simulink model ""  (R2025b)
settings: Solver=FixedStepAuto  StartTime=0.0  StopTime=inf  FixedStep=.02  RelTol=1e-3
libraries: simulink x3
settings Model: Creator=ajax  LastModifiedBy=ajax

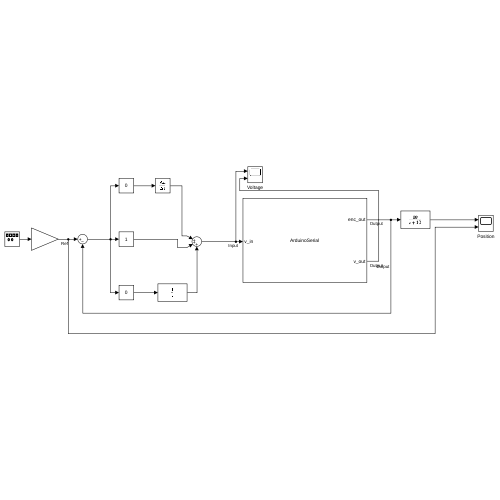
[thumbnail: Simulink's stored preview of the top-level diagram]
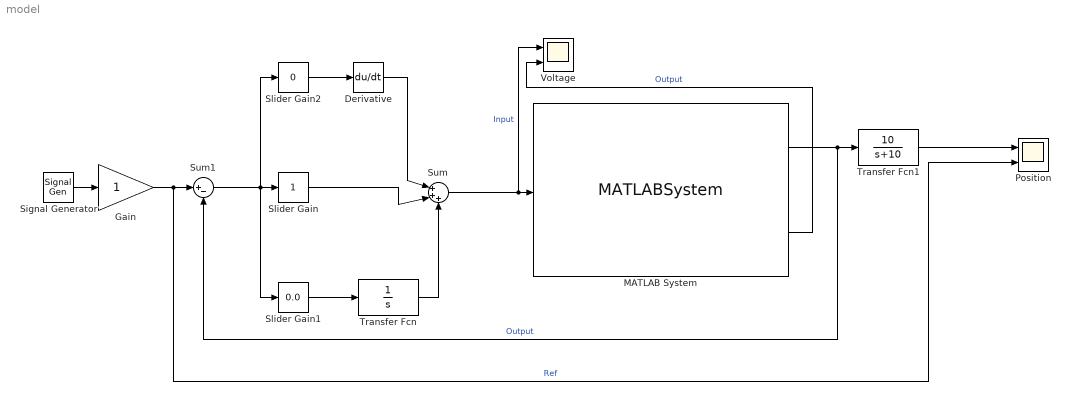
== system model ==
  Derivative : Derivative
  Gain : Gain
  MATLAB System : MATLABSystem  System=ArduinoSerial  COMPort=/dev/ttyACM0  BaudRate=115200  SimulateUsing=Interpreted execution
      mask Type: ArduinoSerial
  Position : Scope  NumInputPorts=2
      settings: ActiveDisplayYMinimum=-12131.749999999998  ActiveDisplayYMaximum=109165.75
  Signal Generator : SignalGenerator  WaveForm=square  Frequency=.5
  Slider Gain : simulink/Math Operations/Slider Gain  gain=1  low=0  high=2
  Slider Gain1 : simulink/Math Operations/Slider Gain  gain=0.0  low=0  high=2
  Slider Gain2 : simulink/Math Operations/Slider Gain  gain=0  low=0  high=2
  Sum : Sum  Inputs=|+++
  Sum1 : Sum  Inputs=|+-
  Transfer Fcn : TransferFcn  Denominator=[1 0]
  Transfer Fcn1 : TransferFcn  Numerator=[10]  Denominator=[1 10]
  Voltage : Scope  NumInputPorts=2
      settings: ActiveDisplayYMinimum=-108237.6717  ActiveDisplayYMaximum=3759.045299999998
  wires:
  Slider Gain2/1 -> Derivative/1
  Derivative/1 -> Sum/1
  Slider Gain/1 -> Sum/2
  Slider Gain1/1 -> Transfer Fcn/1
  Transfer Fcn/1 -> Sum/3
  MATLAB System/1 -> Transfer Fcn1/1, Sum1/2  "Output"
  Signal Generator/1 -> Gain/1
  Gain/1 -> Position/2, Sum1/1  "Ref"
  Sum/1 -> Voltage/1, MATLAB System/1  "Input"
  MATLAB System/2 -> Voltage/2  "Output"
  Sum1/1 -> Slider Gain2/1, Slider Gain1/1, Slider Gain/1
  Transfer Fcn1/1 -> Position/1
